simulink library "Gear_Stage"  (R2018b)
settings: Solver=VariableStepAuto  StartTime=0.0  StopTime=10.0  RelTol=1e-3
settings Model: Creator=Alexander Koch  LastModifiedBy=ga69qig
settings SFSimCC: SimUseLocalCustomCode=off
settings RTWCC: RTWUseLocalCustomCode=off
settings CodeAppCC: StateflowObjectComments=on

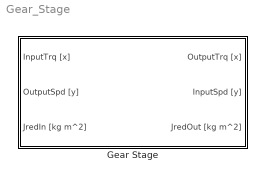
== system Gear_Stage ==
  Gear Stage : Subsystem  mask(SB){iGear=-5, eta=0.98, JredGetr=0.19, LocalSampleTime=-1}
      mask prompts: iGear "Gear Ratio [-]"; eta "Efficiency [-]"; JredGetr "Reduced Moment of Inertia [kg m^2]"; LocalSampleTime "Local System Sample-Time [s]"
      mask help:
      | <Author> Alexander Koch [1]</Author>
      | <Date> 09/03/2017 </Date>
      |
      | <Description>
      | Requires input torque, input revolution speed, gear ratio and efficiency and calculates output torque and revoultion speed. Gear ratio is defined by i=InputSpd/OutputSpd. Efficiency reduces output Torque. To represent the revolution and torque direction of one stage, i has to be negative.
      | </Description>
      mask init:
      | GlobalSampleTime = CalcGlobalSampleTime(LocalSampleTime);
      mask Help:
      | <Parameters>
      | Efficiency [-]
      | Gear Ratio [-]
      | Reduced Moment of Inertia [kg m^2]
      | Local System Sample-Time [s]
      | 	<Min> GlobalSampleTime </Min>
      | Global Sample-Time [s]
      | </Parameters>
      | 
      | <Inputs>
      | InputTrq [x]
      | InputSpd [y]
      | </Inputs>
      | 
      | <Outputs>
      | OutputTrq [x]
      | OutputSpd [y]
      | </Outputs>
      | <Sources>
      | [1] B. Danquah, A. Koch, A. Pinnel, and M. Lienkamp, “Modular, Open Source Simulation Approach: Application to Design and Analyze Electric Vehicles,” in 2019 Fourteenth International Conference on Ecological Vehicles and Renewable Energies, Monaco, 2019, pp. 1–8.
      | </Sources>
      mask TypeOptions iGear:
      | Uebersetzung
      | /Value
      mask TypeOptions eta:
      | Wirkungsgrad
      | /Value
      mask TypeOptions LocalSampleTime:
      | InputTrq [x]/SampleTime | OutputSpd [y]
      | 
      | /SampleTime | JredIn [kg m^2]/SampleTime
      mask DialogControl Container3 Prompt: Documentation:
      mask DialogControl Control2 Prompt: %<MaskHelp>
      mask DialogControl Container5 Prompt: Sample Time
      mask Display:
      | [picturexpos,pictureypos,picturewidth,pictureheight] = ...
      |     CalcBlockPicturePosition(gcb,1,0.01,0.1,80,80); % calculating picture position depending on Block size and minimum margin size
      | image('Gear_Stage.svg',[picturexpos pictureypos picturewidth pictureheight]); % plot picture to block

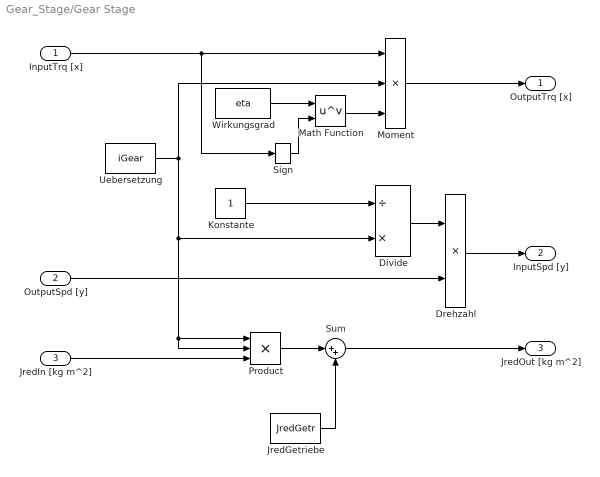
== system Gear_Stage/Gear Stage ==
  InputTrq [x] : Inport  SampleTime=LocalSampleTime
  "OutputSpd [y] " : Inport  Port=2  SampleTime=LocalSampleTime
  JredIn [kg m^2] : Inport  Port=3  SampleTime=LocalSampleTime
  Divide : Product  Inputs=/*
  Drehzahl : Product
  JredGetriebe : Constant  Value=JredGetr
  Konstante : Constant
  Math Function : Math  Operator=pow  SaturateOnIntegerOverflow=on
  Moment : Product  Inputs=3
  Product : Product  Inputs=3
  Sign : Signum
  Sum : Sum  Inputs=|++
  "Uebersetzung " : Constant  Value=iGear
  "Wirkungsgrad " : Constant  Value=eta
  OutputTrq [x] : Outport  SampleTime=GlobalSampleTime
  InputSpd [y] : Outport  Port=2  SampleTime=GlobalSampleTime
  JredOut [kg m^2] : Outport  Port=3  SampleTime=GlobalSampleTime
  wires:
  Divide/1 -> Drehzahl/1
  InputTrq [x]/1 -> Sign/1, Moment/1
  "OutputSpd [y] "/1 -> Drehzahl/2
  Konstante/1 -> Divide/1
  Moment/1 -> OutputTrq [x]/1
  Drehzahl/1 -> InputSpd [y]/1
  "Uebersetzung "/1 -> Moment/2, Product/2, Product/1, Divide/2
  "Wirkungsgrad "/1 -> Math Function/1
  Math Function/1 -> Moment/3
  Sign/1 -> Math Function/2
  JredIn [kg m^2]/1 -> Product/3
  Product/1 -> Sum/1
  Sum/1 -> JredOut [kg m^2]/1
  JredGetriebe/1 -> Sum/2
